simulink model "FOC_BLDC_HIL"  (R2021a)
settings: Solver=FixedStepDiscrete  StartTime=0.0  StopTime=2  RelTol=1e-3  EnableMultiTasking=on
undefined symbols (not defined in the file): DiscIntNeverNeededParam, Init_angle, J, Kawspeed, Ke, Kspeed, Lsx, Lsy, negVid, negVTm, oversampling, p, posVid, posVTm, Psim, Rs, T_load, Ts, ts_FPGA_clk, ts_FPGA_mdl, Ts_svpwm, Tsp, Vdc, Viq, VTm
libraries: simulink x93, hdlsllib x23, slrealtimeloglib x3
(part 3 of 4)

== system FOC_BLDC_HIL/Field Oriented Control ==
  Wm_ref : Inport
  Mech_Speed : Inport  Port=2
  iabc : Inport  Port=3
  Angle estimation : Subsystem
  Clark and Park Transform : Subsystem
  Current Controller : Subsystem
  Rate Transition1 : RateTransition  OutPortSampleTime=Tsp
  Rate Transition7 : RateTransition  OutPortSampleTime=Ts
  SVPWM : Subsystem
  Speed Controller : Subsystem
  "rpm -> rad/s [mech.]" : Gain  Gain=2*pi/60
  Ta,Tb,Tc : Outport
  wires:
  Speed Controller/1(idq_ref) -> Rate Transition7/1
  Wm_ref/1 -> "rpm -> rad/s [mech.]"/1
  Rate Transition1/1 -> Speed Controller/2(Wm)
  iabc/1 -> Clark and Park Transform/2(iabc)
  Mech_Speed/1 -> Angle estimation/1(Mech_Speed), Rate Transition1/1, Current Controller/3(Wm)
  Current Controller/1(vabc*) -> SVPWM/1(vabc*)
  Rate Transition7/1 -> Current Controller/1(Idq_ref)
  Clark and Park Transform/1(idq) -> Current Controller/2(idq)
  "rpm -> rad/s [mech.]"/1 -> Speed Controller/1(Wm_ref)
  SVPWM/1("Ta,Tb,Tc ") -> Ta,Tb,Tc/1
  Angle estimation/1(angle_el) -> Current Controller/4(Angle_el), Clark and Park Transform/1(angle)

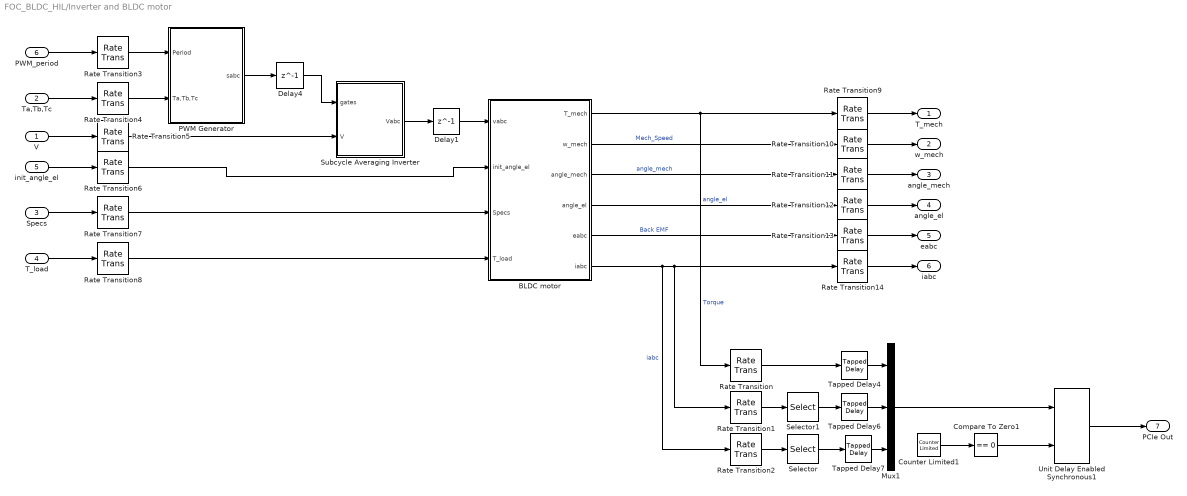
== system FOC_BLDC_HIL/Inverter and BLDC motor ==
  V : Inport
  Ta,Tb,Tc : Inport  Port=2
  Specs : Inport  Port=3
  T_load : Inport  Port=4
  init_angle_el : Inport  Port=5
  PWM_period : Inport  Port=6
  "\tPWM Generator" : Subsystem
  BLDC motor : Subsystem
  Compare To Zero1 : simulink/Logic and Bit Operations/Compare To Zero  relop===  OutDataTypeStr=boolean
  Counter Limited1 : simulink/Sources/Counter Limited  uplimit=49  tsamp=Ts
  Delay1 : Delay  DelayLength=1
  Delay4 : Delay  DelayLength=1
  Mux1 : Mux  Inputs=3
  Rate Transition{,1..2,5..8,10} (8 alike) : RateTransition
  Rate Transition{9,11..14} (5 alike) : RateTransition  OutPortSampleTime=Ts
  Rate Transition3 : RateTransition  OutPortSampleTime=ts_FPGA_clk
  Rate Transition4 : RateTransition  OutPortSampleTime=ts_FPGA_clk
  Selector : Selector  InputPortWidth=3  IndexOptions=Index vector (dialog)  Indices=[2]  OutputSizes=1
  Selector1 : Selector  InputPortWidth=3  IndexOptions=Index vector (dialog)  Indices=[1]  OutputSizes=1
  Subcycle Averaging Inverter : Subsystem
  Tapped Delay4 : simulink/Discrete/Tapped Delay  vinit=0.0  samptime=Ts  NumDelays=50  DelayOrder=Oldest  includeCurrent=off
  Tapped Delay6 : simulink/Discrete/Tapped Delay  vinit=0.0  samptime=Ts  NumDelays=50  DelayOrder=Oldest  includeCurrent=off
  Tapped Delay7 : simulink/Discrete/Tapped Delay  vinit=0.0  samptime=Ts  NumDelays=50  DelayOrder=Oldest  includeCurrent=off
  Unit Delay Enabled Synchronous1 : hdlsllib/Discrete/Unit Delay Enabled Synchronous  InitialCondition=0.0  SampleTime=Ts
      settings: SourceProductName=HDL Coder
  T_mech : Outport
  w_mech : Outport  Port=2
  angle_mech : Outport  Port=3
  angle_el : Outport  Port=4
  eabc : Outport  Port=5
  iabc : Outport  Port=6
  PCIe Out : Outport  Port=7
  wires:
  BLDC motor/3(angle_mech) -> Rate Transition11/1  "angle_mech"
  BLDC motor/5(eabc) -> Rate Transition13/1  "Back EMF"
  Ta,Tb,Tc/1 -> Rate Transition4/1
  PWM_period/1 -> Rate Transition3/1
  "\tPWM Generator"/1("sabc ") -> Delay4/1
  Subcycle Averaging Inverter/1(Vabc) -> Delay1/1
  init_angle_el/1 -> Rate Transition6/1
  Specs/1 -> Rate Transition7/1
  T_load/1 -> Rate Transition8/1
  Delay4/1 -> Subcycle Averaging Inverter/1(gates)
  V/1 -> Rate Transition5/1
  Delay1/1 -> BLDC motor/1(vabc)
  Tapped Delay4/1 -> Mux1/1
  Compare To Zero1/1 -> Unit Delay Enabled Synchronous1/2
  Unit Delay Enabled Synchronous1/1 -> PCIe Out/1
  Mux1/1 -> Unit Delay Enabled Synchronous1/1
  BLDC motor/1(T_mech) -> Rate Transition/1, Rate Transition9/1  "Torque"
  BLDC motor/6(iabc) -> Rate Transition2/1, Rate Transition1/1, Rate Transition14/1  "iabc"
  BLDC motor/4(angle_el) -> Rate Transition12/1  "angle_el"
  BLDC motor/2(w_mech) -> Rate Transition10/1  "Mech_Speed"
  Counter Limited1/1 -> Compare To Zero1/1
  Selector/1 -> Tapped Delay7/1
  Tapped Delay6/1 -> Mux1/2
  Tapped Delay7/1 -> Mux1/3
  Selector1/1 -> Tapped Delay6/1
  Rate Transition2/1 -> Selector/1
  Rate Transition1/1 -> Selector1/1
  Rate Transition/1 -> Tapped Delay4/1
  Rate Transition3/1 -> "\tPWM Generator"/1(Period)
  Rate Transition4/1 -> "\tPWM Generator"/2(Ta,Tb,Tc)
  Rate Transition5/1 -> Subcycle Averaging Inverter/2(V)
  Rate Transition6/1 -> BLDC motor/2(init_angle_el)
  Rate Transition7/1 -> BLDC motor/3(Specs)
  Rate Transition8/1 -> BLDC motor/4(T_load)
  Rate Transition9/1 -> T_mech/1
  Rate Transition10/1 -> w_mech/1
  Rate Transition11/1 -> angle_mech/1
  Rate Transition12/1 -> angle_el/1
  Rate Transition13/1 -> eabc/1
  Rate Transition14/1 -> iabc/1

== system FOC_BLDC_HIL/Motor Specifications ==
  Data Type Conversion11 : DataTypeConversion  OutDataTypeStr=single  RndMeth=Nearest
  Moment of inertia reciprocal : Constant  Value=1/J  SampleTime=-1
  Mux : Mux  Inputs=7
  Number of pole pairs : Constant  Value=p  SampleTime=Ts
  Permanent magnetic flux linkage : Constant  Value=Psim  SampleTime=-1
  Reciprocal : Product  Inputs=/
  Stator Resistance : Constant  Value=Rs  SampleTime=-1
  Stator inductance in d-axis reciprocal : Constant  Value=1/Lsx  SampleTime=-1
  Stator inductance in q-axis reciprocal : Constant  Value=1/Lsy  SampleTime=-1
  Specs : Outport
  wires:
  Stator inductance in q-axis reciprocal/1 -> Mux/7
  Number of pole pairs/1 -> Reciprocal/1, Mux/1
  Stator inductance in d-axis reciprocal/1 -> Mux/6
  Permanent magnetic flux linkage/1 -> Mux/3
  Stator Resistance/1 -> Mux/5
  Mux/1 -> Data Type Conversion11/1
  Data Type Conversion11/1 -> Specs/1
  Moment of inertia reciprocal/1 -> Mux/4
  Reciprocal/1 -> Mux/2

== system FOC_BLDC_HIL/Subsystem1 ==
  Torque : Inport
  Mech_Speed : Inport  Port=2
  angle_mech : Inport  Port=3
  angle_el : Inport  Port=4
  Back EMF : Inport  Port=5
  iabc : Inport  Port=6
  tag scope: Angle_el=global, Angle_m=global, Iabc=global, Speed=global, Torque=global, back_emf=global
  wires:
  Torque/1 -> [Torque]
  Mech_Speed/1 -> [Speed]
  Back EMF/1 -> [back_emf]
  angle_mech/1 -> [Angle_m]
  iabc/1 -> [Iabc]
  angle_el/1 -> [Angle_el]

== system FOC_BLDC_HIL/Field Oriented Control/Angle estimation ==
  Mech_Speed : Inport
  Discrete-Time Integrator1 : DiscreteIntegrator  SampleTime=-1  ICPrevOutput=DiscIntNeverNeededParam  ICPrevScaledInput=DiscIntNeverNeededParam
  Initial motor angle : Constant  Value=Init_angle  OutDataTypeStr=single
  Sum4 : Sum  OutDataTypeStr=single
  Wrapped Discrete Time Integrator : Subsystem
  p/2 : Gain  Gain=p
  angle_el : Outport
  wires:
  p/2/1 -> Wrapped Discrete Time Integrator/1(In1)  "electrical_speed"
  Wrapped Discrete Time Integrator/1(Out1) -> Sum4/1
  Mech_Speed/1 -> p/2/1
  Sum4/1 -> angle_el/1  "Electrical_angle"
  Initial motor angle/1 -> Sum4/2

== system FOC_BLDC_HIL/Field Oriented Control/Clark and Park Transform ==
  angle : Inport
  iabc : Inport  Port=2
  Phase advancement : Subsystem  Commented=on
  Sine_Cosine : Trigonometry  Operator=sincos
  "abc -> d/q" : Subsystem
  idq : Outport  VectorParamsAs1DForOutWhenUnconnected=off
  wires:
  Sine_Cosine/1 -> "abc -> d/q"/2(Sin)
  Sine_Cosine/2 -> "abc -> d/q"/3(Cos)
  iabc/1 -> "abc -> d/q"/1(iabc)
  "abc -> d/q"/1(idq) -> idq/1
  angle/1 -> Sine_Cosine/1

== system FOC_BLDC_HIL/Field Oriented Control/Current Controller ==
  Idq_ref : Inport
  idq : Inport  Port=2
  Wm : Inport  Port=3
  Angle_el : Inport  Port=4
  Phase advancement : Subsystem
  Sine_Cosine : Trigonometry  Operator=sincos
  Trapezoidal emf estimator : Subsystem
  "d/q -> abc" : Subsystem
  d/q controller : Subsystem
  vabc* : Outport  VectorParamsAs1DForOutWhenUnconnected=off
  wires:
  Trapezoidal emf estimator/1(Trapezoidal edq) -> d/q controller/3(edq)
  Idq_ref/1 -> d/q controller/1(Idq_ref)
  idq/1 -> d/q controller/2(idq)
  Angle_el/1 -> Trapezoidal emf estimator/2(Angle_el), Phase advancement/1(angle)
  Wm/1 -> Trapezoidal emf estimator/1(Wm)
  Sine_Cosine/1 -> "d/q -> abc"/2(Sin)
  Sine_Cosine/2 -> "d/q -> abc"/3(Cos)
  Phase advancement/1(ph.adv. angle) -> Sine_Cosine/1
  d/q controller/1(vdq) -> "d/q -> abc"/1(vdq)
  "d/q -> abc"/1(vabc) -> vabc*/1

== system FOC_BLDC_HIL/Field Oriented Control/SVPWM ==
  vabc* : Inport
  Application times : Subsystem
  Magnitude Invariant Clark : Subsystem
  On-state times : Subsystem
  Sector selector : Subsystem
  Ts_svpwm : Constant  Value=Ts_svpwm  OutDataTypeStr=single
  Vdc : Constant  Value=Vdc  OutDataTypeStr=single  SampleTime=-1
  XYZ : Subsystem
  "Ta,Tb,Tc " : Outport  VectorParamsAs1DForOutWhenUnconnected=off
  wires:
  Ts_svpwm/1 -> Application times/3(Ts), On-state times/3(Ts), XYZ/3(Ts)
  Sector selector/1(N) -> On-state times/1(N), Application times/1(N)
  Application times/1(T1,T2) -> On-state times/2("T1,T2 ")
  Magnitude Invariant Clark/1(Valphabeta) -> Sector selector/1(Valphabeta), XYZ/2(vAB)
  vabc*/1 -> Magnitude Invariant Clark/1(vabc)
  XYZ/1(XYZ) -> Application times/2(XYZ)
  Vdc/1 -> XYZ/1(VDC)
  On-state times/1(Ta,Tb,Tc) -> "Ta,Tb,Tc "/1

== system FOC_BLDC_HIL/Field Oriented Control/Speed Controller ==
  Wm_ref : Inport
  Wm : Inport  Port=2
  Speed controller : Subsystem
  idq_ref : Outport  VectorParamsAs1DForOutWhenUnconnected=off
  wires:
  Wm_ref/1 -> Speed controller/1(Wm_ref)
  Wm/1 -> Speed controller/2(Wm)
  Speed controller/1(idq_ref) -> idq_ref/1

== system FOC_BLDC_HIL/Inverter and BLDC motor/	PWM Generator ==
  Period : Inport
  Ta,Tb,Tc : Inport  Port=2
  Demux : Demux  Outputs=3
  Logical Operator : Logic  Operator=NOT  AllPortsSameDT=off  OutDataTypeStr=boolean
  Logical Operator1 : Logic  Operator=NOT  AllPortsSameDT=off  OutDataTypeStr=boolean
  Logical Operator2 : Logic  Operator=NOT  AllPortsSameDT=off  OutDataTypeStr=boolean
  Mux : Mux  Inputs=6
  Relational Operator1 : RelationalOperator  Operator=>  OutDataTypeStr=boolean  RndMeth=Nearest
  Relational Operator2 : RelationalOperator  Operator=>  OutDataTypeStr=boolean  RndMeth=Nearest
  Relational Operator3 : RelationalOperator  Operator=>  OutDataTypeStr=boolean  RndMeth=Nearest
  Unit Delay : UnitDelay  SampleTime=-1  HasFrameUpgradeWarning=on
  carrier_wave1 : Subsystem
  "sabc " : Outport  VectorParamsAs1DForOutWhenUnconnected=off
  wires:
  Unit Delay/1 -> Relational Operator3/1, Relational Operator2/1, Relational Operator1/1  "Counter"
  Relational Operator1/1 -> Logical Operator/1, Mux/1  "A"
  Relational Operator2/1 -> Mux/3, Logical Operator1/1  "B"
  Logical Operator1/1 -> Mux/4  "B_"
  Relational Operator3/1 -> Mux/5, Logical Operator2/1  "C"
  Logical Operator2/1 -> Mux/6  "C_"
  Logical Operator/1 -> Mux/2  "A_"
  Mux/1 -> "sabc "/1  "G"
  Demux/1 -> Relational Operator1/2  "A_comp"
  Demux/2 -> Relational Operator2/2  "B_comp"
  Demux/3 -> Relational Operator3/2  "C_comp"
  Ta,Tb,Tc/1 -> Demux/1
  Period/1 -> carrier_wave1/1(PWM_period)
  carrier_wave1/1(counter) -> Unit Delay/1

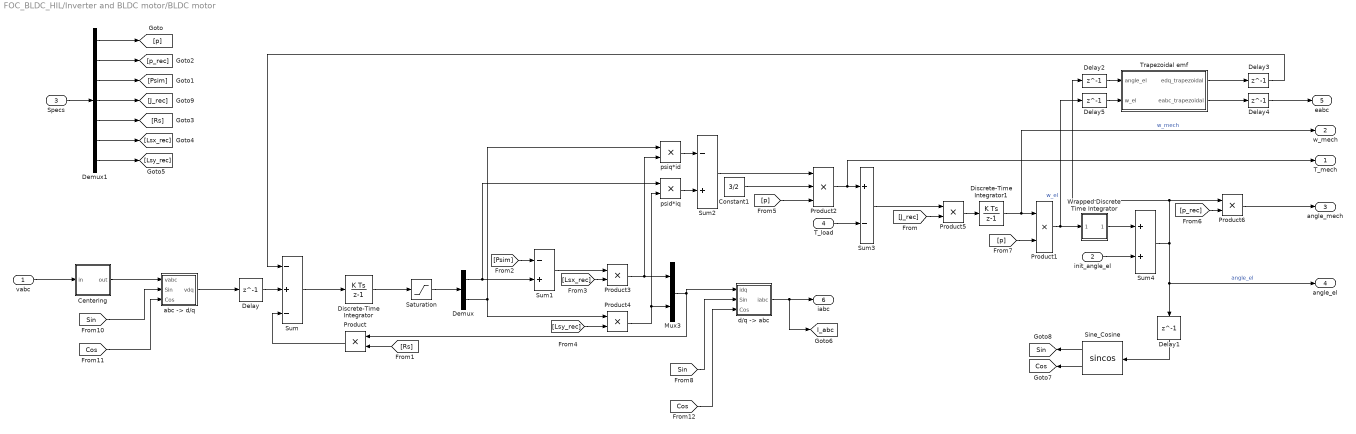
== system FOC_BLDC_HIL/Inverter and BLDC motor/BLDC motor ==
  vabc : Inport
  init_angle_el : Inport  Port=2
  Specs : Inport  Port=3
  T_load : Inport  Port=4
  Centering : Subsystem
  Constant1 : Constant  Value=3/2  OutDataTypeStr=single  SampleTime=-1
  Delay{,1..5} (6 alike) : Delay  DelayLength=1
  Demux : Demux  Outputs=2
  Demux1 : Demux  Outputs=7
  Discrete-Time Integrator : DiscreteIntegrator  InitialCondition=[Psim 0]'  SampleTime=-1  ICPrevOutput=DiscIntNeverNeededParam  ICPrevScaledInput=DiscIntNeverNeededParam
  Discrete-Time Integrator1 : DiscreteIntegrator  SampleTime=-1  ICPrevOutput=DiscIntNeverNeededParam  ICPrevScaledInput=DiscIntNeverNeededParam
  Mux3 : Mux  Inputs=2
  Product{,1,3..6} (6 alike) : Product
  Product2 : Product  Inputs=3
  Saturation : Saturate  UpperLimit=2*[Psim Psim]'  LowerLimit=-2*[Psim Psim]'
  Sine_Cosine : Trigonometry  Operator=sincos
  Sum : Sum  Inputs=-+-
  Sum1 : Sum  Inputs=-+
  Sum2 : Sum  Inputs=-+
  Sum3 : Sum  Inputs=+-
  Sum4 : Sum  OutDataTypeStr=single
  Trapezoidal emf : Subsystem
  Wrapped Discrete Time Integrator : Subsystem
  "abc -> d/q" : Subsystem
  "d/q -> abc" : Subsystem
  psid*iq : Product
  psiq*id : Product
  T_mech : Outport  VectorParamsAs1DForOutWhenUnconnected=off
  w_mech : Outport  Port=2  VectorParamsAs1DForOutWhenUnconnected=off
  angle_mech : Outport  Port=3  VectorParamsAs1DForOutWhenUnconnected=off
  angle_el : Outport  Port=4  VectorParamsAs1DForOutWhenUnconnected=off
  eabc : Outport  Port=5  VectorParamsAs1DForOutWhenUnconnected=off
  iabc : Outport  Port=6  VectorParamsAs1DForOutWhenUnconnected=off
  tag scope: Cos=global, I_abc=global, Sin=global
  wires:
  Product4/1 -> psid*iq/2, Mux3/2
  [Psim] -> Sum1/1
  psiq*id/1 -> Sum2/1
  Product3/1 -> Mux3/1, psiq*id/2
  Mux3/1 -> "d/q -> abc"/1(idq), Product/1
  psid*iq/1 -> Sum2/2
  Sum/1 -> Discrete-Time Integrator/1
  T_load/1 -> Sum3/2
  Demux/1 -> Sum1/2, psid*iq/1
  Sum1/1 -> Product3/1
  Product5/1 -> Discrete-Time Integrator1/1
  Demux/2 -> Product4/1, psiq*id/1
  Discrete-Time Integrator1/1 -> w_mech/1, Product1/1  "w_mech"
  Product2/1 -> T_mech/1, Sum3/1
  Discrete-Time Integrator/1 -> Saturation/1
  Product6/1 -> angle_mech/1
  Saturation/1 -> Demux/1
  Wrapped Discrete Time Integrator/1(Out1) -> Sum4/1
  init_angle_el/1 -> Sum4/2
  Sum4/1 -> Product6/1, Delay2/1, Delay1/1, angle_el/1  "angle_el"
  Product1/1 -> Wrapped Discrete Time Integrator/1(In1), Delay5/1  "w_el"
  Specs/1 -> Demux1/1
  Product/1 -> Sum/3
  [Rs] -> Product/2
  [Lsx_rec] -> Product3/2
  [Lsy_rec] -> Product4/2
  Sum2/1 -> Product2/1
  Constant1/1 -> Product2/2
  [p] -> Product2/3
  Sum3/1 -> Product5/1
  [J_rec] -> Product5/2
  [p] -> Product1/2
  Demux1/1 -> [p]
  Demux1/5 -> [Rs]
  Demux1/6 -> [Lsx_rec]
  Demux1/7 -> [Lsy_rec]
  Demux1/2 -> [p_rec]
  Trapezoidal emf/1(edq_trapezoidal) -> Delay3/1
  Trapezoidal emf/2(eabc_trapezoidal) -> Delay4/1
  Sine_Cosine/2 -> [Cos]
  Sine_Cosine/1 -> [Sin]
  vabc/1 -> Centering/1(in)
  Centering/1(out) -> "abc -> d/q"/1(vabc)
  [Sin] -> "abc -> d/q"/2(Sin)
  [Cos] -> "abc -> d/q"/3(Cos)
  "abc -> d/q"/1(vdq) -> Delay/1
  "d/q -> abc"/1(iabc) -> [I_abc], iabc/1
  [Sin] -> "d/q -> abc"/2(Sin)
  [Cos] -> "d/q -> abc"/3(Cos)
  Delay/1 -> Sum/2
  Delay1/1 -> Sine_Cosine/1
  Delay2/1 -> Trapezoidal emf/1(angle_el)
  Delay3/1 -> Sum/1
  Delay4/1 -> eabc/1
  Delay5/1 -> Trapezoidal emf/2(w_el)
  Demux1/4 -> [J_rec]
  Demux1/3 -> [Psim]
  [p_rec] -> Product6/2

== system FOC_BLDC_HIL/Inverter and BLDC motor/Subcycle Averaging Inverter ==
  gates : Inport
  V : Inport  Port=2
  Constant2 : Constant  Value=0  OutDataTypeStr=uint32  SampleTime=1e-6
  Constant3 : Constant  Value=false  SampleTime=-1
  Gain : Gain  Gain=-1
  Inverter (2-Level HDL w faults) : Subsystem  mask{rSnub=10000, rSwitch=0.001, vfSwitch=0, rDiode=0.001, vfDiode=0.8}
      mask prompts: rSnub "Snubber Resistance (Ohms)"; rSwitch "Switch Resistance (Ohms)"; vfSwitch "Switch Forward Voltage (V)"; rDiode "Diode Resistance (Ohms)"; vfDiode "Diode Forward Voltage (V)"
  Selector : Selector  InputPortWidth=3  IndexOptions=Index vector (dialog)  Indices=[1 2]  OutputSizes=1
  Terminator : Terminator
  Terminator1 : Terminator
  Vabc : Outport
  wires:
  Gain/1 -> Inverter (2-Level HDL w faults)/4(V_minus)
  Constant3/1 -> Inverter (2-Level HDL w faults)/6(ideal_switch_flag)
  V/1 -> Inverter (2-Level HDL w faults)/3(V_plus), Gain/1
  Constant2/1 -> Inverter (2-Level HDL w faults)/5(Fault_Word)
  Inverter (2-Level HDL w faults)/3(IDC) -> Terminator1/1
  [I_abc] -> Inverter (2-Level HDL w faults)/2(Iout)
  gates/1 -> Inverter (2-Level HDL w faults)/1(Gates)
  Inverter (2-Level HDL w faults)/1(Vll) -> Selector/1
  Inverter (2-Level HDL w faults)/2(V) -> Vabc/1
  Selector/1 -> Terminator/1

== system FOC_BLDC_HIL/Field Oriented Control/Angle estimation/Wrapped Discrete Time Integrator ==
  In1 : Inport
  Add1 : Sum  Inputs=+++
  Compare To Constant1 : simulink/Logic and Bit Operations/Compare To Constant  relop=>=  const=2*pi  OutDataTypeStr=boolean
  Compare To Constant2 : simulink/Logic and Bit Operations/Compare To Constant  relop=<  const=0  OutDataTypeStr=boolean
  Constant2 : Constant  Value=-2*pi  OutDataTypeStr=single  SampleTime=-1
  Constant3 : Constant  Value=2*pi  OutDataTypeStr=single  SampleTime=-1
  Constant5 : Constant  Value=0  OutDataTypeStr=single  SampleTime=-1
  Gain : Gain  Gain=Ts
  Switch2 : Switch  Criteria=u2 ~= 0
  Switch3 : Switch  Criteria=u2 ~= 0
  Unit Delay : UnitDelay  SampleTime=-1  HasFrameUpgradeWarning=on
  Out1 : Outport  VectorParamsAs1DForOutWhenUnconnected=off
  wires:
  Add1/1 -> Unit Delay/1
  In1/1 -> Gain/1
  Unit Delay/1 -> Out1/1, Add1/1, Compare To Constant2/1, Compare To Constant1/1
  Compare To Constant1/1 -> Switch3/2
  Compare To Constant2/1 -> Switch2/2
  Constant3/1 -> Switch2/1
  Constant5/1 -> Switch2/3
  Switch2/1 -> Switch3/3
  Constant2/1 -> Switch3/1
  Switch3/1 -> Add1/3
  Gain/1 -> Add1/2

== system FOC_BLDC_HIL/Field Oriented Control/Clark and Park Transform/Phase advancement ==
  angle : Inport
  Discrete Derivative : simulink/Discrete/Discrete Derivative  gainval=1.0  ICPrevScaledInput=0.0  OutMin=[]  OutMax=[]  OutDataType=fixdt(1, 16)  OutScaling=2^-10  DoSatur=off
  Sum2 : Sum
  Ts : Gain  Gain=Ts
  ph.adv. angle : Outport  VectorParamsAs1DForOutWhenUnconnected=off
  wires:
  Sum2/1 -> ph.adv. angle/1
  Ts/1 -> Sum2/1
  angle/1 -> Discrete Derivative/1, Sum2/2
  Discrete Derivative/1 -> Ts/1

== system FOC_BLDC_HIL/Field Oriented Control/Clark and Park Transform/abc -> d//q ==
  iabc : Inport
  Sin : Inport  Port=2
  Cos : Inport  Port=3
  Demux : Demux  Outputs=3
  Gain : Gain  Gain=sqrt(3/2)
  Gain1 : Gain  Gain=sqrt(1/2)
  Gain2 : Gain  Gain=-1  OutDataTypeStr=single
  Mux2 : Mux  Inputs=2
  Product{,1..3} (4 alike) : Product
  Subtract : Sum  Inputs=+-
  Subtract1 : Sum
  Sum : Sum  Inputs=+|-
  idq : Outport  VectorParamsAs1DForOutWhenUnconnected=off
  wires:
  iabc/1 -> Demux/1
  Demux/1 -> Gain/1
  Demux/2 -> Sum/1
  Demux/3 -> Sum/2
  Gain/1 -> Product2/1, Product/1  "Alpha"
  Mux2/1 -> idq/1
  Sum/1 -> Gain1/1
  Cos/1 -> Product3/2, Product/2
  Gain1/1 -> Product3/1, Product1/1  "Beta"
  Sin/1 -> Gain2/1
  Product/1 -> Subtract/1
  Product1/1 -> Subtract/2
  Subtract/1 -> Mux2/1
  Product2/1 -> Subtract1/1
  Product3/1 -> Subtract1/2
  Subtract1/1 -> Mux2/2
  Gain2/1 -> Product1/2, Product2/2

== system FOC_BLDC_HIL/Field Oriented Control/Current Controller/Phase advancement ==
  angle : Inport
  Discrete Derivative : simulink/Discrete/Discrete Derivative  gainval=1.0  ICPrevScaledInput=0.0  OutMin=[]  OutMax=[]  OutDataType=fixdt(1, 16)  OutScaling=2^-10  DoSatur=off
  Sum2 : Sum
  Ts : Gain  Gain=Ts
  ph.adv. angle : Outport  VectorParamsAs1DForOutWhenUnconnected=off
  wires:
  Sum2/1 -> ph.adv. angle/1
  Ts/1 -> Sum2/1
  angle/1 -> Discrete Derivative/1, Sum2/2
  Discrete Derivative/1 -> Ts/1

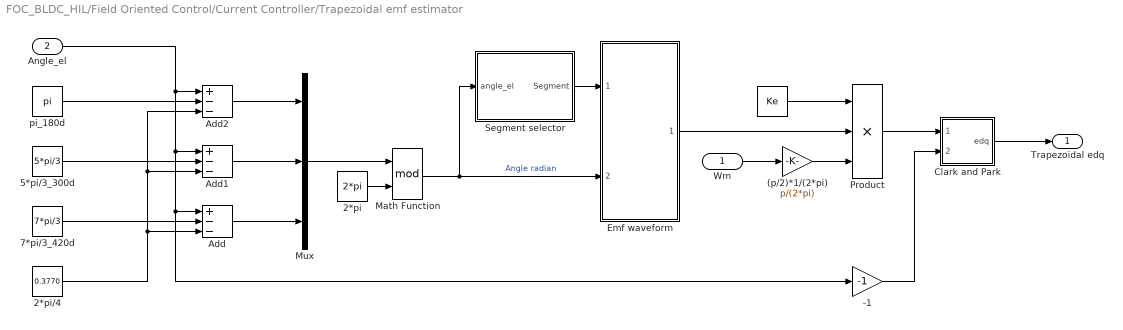
== system FOC_BLDC_HIL/Field Oriented Control/Current Controller/Trapezoidal emf estimator ==
  Wm : Inport
  Angle_el : Inport  Port=2
  "  " : Constant  Value=Ke  OutDataTypeStr=single  SampleTime=-1
  "  Add2" : Sum  Inputs=+--
  " Add1 " : Sum  Inputs=+--
  (p/2)*1/(2*pi) : Gain  Gain=p/(2*pi)
  -1 : Gain  Gain=-1
  2*pi : Constant  Value=2*pi  OutDataTypeStr=single  SampleTime=-1
  2*pi/4 : Constant  Value=0.3770  OutDataTypeStr=single  SampleTime=-1
  5*pi/3_300d : Constant  Value=5*pi/3  OutDataTypeStr=single  SampleTime=-1
  7*pi/3_420d : Constant  Value=7*pi/3  OutDataTypeStr=single  SampleTime=-1
  "Add " : Sum  Inputs=+--
  Clark and Park : Subsystem
  Emf waveform : Subsystem
  Math Function : Math  Operator=mod  SignedPower=on  SaturateOnIntegerOverflow=on
  Mux : Mux  Inputs=3
  Product : Product  Inputs=3
  Segment selector : Subsystem
  pi_180d : Constant  Value=pi  OutDataTypeStr=single  SampleTime=-1
  Trapezoidal edq : Outport  VectorParamsAs1DForOutWhenUnconnected=off
  wires:
  Math Function/1 -> Segment selector/1(angle_el), Emf waveform/2(angle_el)  "Angle radian"
  2*pi/1 -> Math Function/2
  Segment selector/1(Segment) -> Emf waveform/1(Segment)
  " Add1 "/1 -> Mux/2
  5*pi/3_300d/1 -> " Add1 "/2
  "Add "/1 -> Mux/3
  7*pi/3_420d/1 -> "Add "/2
  "  "/1 -> Product/1
  Emf waveform/1(Emf waveform) -> Product/2
  Product/1 -> Clark and Park/1(eabc)
  Wm/1 -> (p/2)*1/(2*pi)/1
  Mux/1 -> Math Function/1
  (p/2)*1/(2*pi)/1 -> Product/3
  -1/1 -> Clark and Park/2(angle)
  Clark and Park/1(edq) -> Trapezoidal edq/1
  "  Add2"/1 -> Mux/1
  pi_180d/1 -> "  Add2"/2
  2*pi/4/1 -> "Add "/3, " Add1 "/3, "  Add2"/3
  Angle_el/1 -> -1/1, "Add "/1, " Add1 "/1, "  Add2"/1

== system FOC_BLDC_HIL/Field Oriented Control/Current Controller/d//q -> abc ==
  vdq : Inport
  Sin : Inport  Port=2
  Cos : Inport  Port=3
  Demux : Demux  Outputs=2
  Gain : Gain  Gain=sqrt(2/3)
  Gain1 : Gain  Gain=-sqrt(1/6)
  Gain2 : Gain  Gain=sqrt(1/2)
  Gain3 : Gain  Gain=sqrt(1/6)
  Gain4 : Gain  Gain=sqrt(1/2)
  Mux2 : Mux  Inputs=3
  Product{,1..3} (4 alike) : Product
  Sum : Sum  Inputs=+|-
  Sum1 : Sum  Inputs=+|+
  Sum2 : Sum  Inputs=+|+
  Sum3 : Sum  Inputs=-|-
  vabc : Outport  VectorParamsAs1DForOutWhenUnconnected=off
  wires:
  vdq/1 -> Demux/1
  Mux2/1 -> vabc/1
  Demux/1 -> Product2/1, Product/1
  Demux/2 -> Product3/1, Product1/1
  Cos/1 -> Product3/2, Product/2
  Sin/1 -> Product2/2, Product1/2
  Product/1 -> Sum/1
  Product1/1 -> Sum/2
  Product3/1 -> Sum1/2
  Product2/1 -> Sum1/1
  Sum/1 -> Gain1/1, Gain3/1, Gain/1  "Alpha"
  Gain/1 -> Mux2/1  "a"
  Gain1/1 -> Sum2/1
  Gain2/1 -> Sum2/2
  Sum1/1 -> Gain4/1, Gain2/1
  Sum2/1 -> Mux2/2  "b"
  Gain3/1 -> Sum3/1
  Gain4/1 -> Sum3/2
  Sum3/1 -> Mux2/3  "c"

== system FOC_BLDC_HIL/Field Oriented Control/Current Controller/d//q controller ==
  Idq_ref : Inport
  idq : Inport  Port=2
  edq : Inport  Port=3
  Demux : Demux  Outputs=2
  Demux1 : Demux  Outputs=2
  Demux2 : Demux  Outputs=2
  Mux1 : Mux  Inputs=2
  Sum1 : Sum  Inputs=+-
  Sum3 : Sum  Inputs=+-
  id controller : Subsystem
  iq controller : Subsystem
  vdq : Outport  VectorParamsAs1DForOutWhenUnconnected=off
  wires:
  Demux/1 -> id controller/2(ed)
  id controller/1(vd) -> Mux1/1
  Demux2/2 -> Sum3/2
  Demux1/2 -> Sum3/1
  Demux/2 -> iq controller/2(eq)
  Sum3/1 -> iq controller/1(iq_error)
  iq controller/1(vq) -> Mux1/2
  Mux1/1 -> vdq/1
  Demux2/1 -> Sum1/2
  Demux1/1 -> Sum1/1
  Sum1/1 -> id controller/1(id_error)
  edq/1 -> Demux/1
  idq/1 -> Demux2/1
  Idq_ref/1 -> Demux1/1

== system FOC_BLDC_HIL/Field Oriented Control/SVPWM/Application times ==
  N : Inport
  XYZ : Inport  Port=2
  Ts : Inport  Port=3
  " " : Gain  Gain=-1
  "  " : Gain  Gain=-1
  "    " : Gain  Gain=-1
  Add : Sum
  Add1 : Sum  Inputs=+--
  Demux : Demux  Outputs=3
  Divide : Product  Inputs=**/
  Divide1 : Product  Inputs=**/
  Multiport Switch : MultiPortSwitch  Inputs=6  DiagnosticForDefault=None
  Multiport Switch1 : MultiPortSwitch  Inputs=6  DiagnosticForDefault=None
  Mux : Mux  Inputs=2
  Switch : Switch
  Switch1 : Switch  Criteria=u2 > Threshold
  T1,T2 : Outport  VectorParamsAs1DForOutWhenUnconnected=off
  wires:
  Demux/2 -> Multiport Switch/3, Multiport Switch1/2, "  "/1
  Demux/3 -> Multiport Switch/2, Multiport Switch1/5, "    "/1
  "    "/1 -> Multiport Switch/4, Multiport Switch1/7
  "  "/1 -> Multiport Switch/7, Multiport Switch1/6
  " "/1 -> Multiport Switch/5, Multiport Switch1/3
  Multiport Switch1/1 -> Switch1/1, Divide1/1, Add/2, Add1/3
  Mux/1 -> T1,T2/1
  Switch/1 -> Mux/1
  Switch1/1 -> Mux/2
  Add/1 -> Divide/3, Divide1/3
  Ts/1 -> Divide1/2, Add1/1, Divide/2
  Multiport Switch/1 -> Add1/2, Add/1, Divide/1, Switch/1
  Divide/1 -> Switch/3
  Add1/1 -> Switch1/2, Switch/2
  Divide1/1 -> Switch1/3
  Demux/1 -> Multiport Switch/6, Multiport Switch1/4, " "/1
  XYZ/1 -> Demux/1
  N/1 -> Multiport Switch1/1, Multiport Switch/1

== system FOC_BLDC_HIL/Field Oriented Control/SVPWM/Magnitude Invariant Clark ==
  vabc : Inport
  "    " : Gain  Gain=sqrt(3)/2
  "     " : Gain  Gain=sqrt(3)/2
  2/3 : Gain  Gain=2/3
  Add1 : Sum  Inputs=+-
  Demux1 : Demux  Outputs=3
  Gain : Gain  Gain=1/2
  Gain1 : Gain  Gain=1/2
  Mux2 : Mux  Inputs=2
  Sum : Sum  Inputs=+--
  Valphabeta : Outport  VectorParamsAs1DForOutWhenUnconnected=off
  wires:
  Demux1/2 -> Gain/1, "     "/1
  Demux1/3 -> Gain1/1, "    "/1
  vabc/1 -> Demux1/1
  "    "/1 -> Add1/2
  "     "/1 -> Add1/1
  Mux2/1 -> 2/3/1
  Add1/1 -> Mux2/2  "Vbeta"
  2/3/1 -> Valphabeta/1
  Gain1/1 -> Sum/3
  Gain/1 -> Sum/2
  Demux1/1 -> Sum/1
  Sum/1 -> Mux2/1  "Valpha"

== system FOC_BLDC_HIL/Field Oriented Control/SVPWM/On-state times ==
  N : Inport
  "T1,T2 " : Inport  Port=2
  Ts : Inport  Port=3
  1/2 : Gain  Gain=1/2
  1/2 also : Gain  Gain=1/2
  1/4 : Gain  Gain=1/4
  Add : Sum  Inputs=+--
  Add1 : Sum
  Add2 : Sum
  Demux2 : Demux  Outputs=2
  Multiport Switch : MultiPortSwitch  Inputs=6  DiagnosticForDefault=None
  Multiport Switch1 : MultiPortSwitch  Inputs=6  DiagnosticForDefault=None
  Multiport Switch2 : MultiPortSwitch  Inputs=6  DiagnosticForDefault=None
  Mux : Mux  Inputs=3
  Ta,Tb,Tc : Outport  VectorParamsAs1DForOutWhenUnconnected=off
  wires:
  "T1,T2 "/1 -> Demux2/1
  Ts/1 -> Add/1
  Demux2/1 -> Add/2, 1/2/1
  Demux2/2 -> Add/3, 1/2 also/1
  Add/1 -> 1/4/1
  1/2/1 -> Add1/2
  1/4/1 -> Add1/1, Multiport Switch2/7, Multiport Switch2/5, Multiport Switch1/6, Multiport Switch1/2, Multiport Switch/4, Multiport Switch/3
  Add1/1 -> Add2/1, Multiport Switch/7, Multiport Switch/2, Multiport Switch2/6, Multiport Switch2/3, Multiport Switch1/5, Multiport Switch1/4
  1/2 also/1 -> Add2/2
  Add2/1 -> Multiport Switch1/3, Multiport Switch/6, Multiport Switch/5, Multiport Switch1/7, Multiport Switch2/2, Multiport Switch2/4
  Multiport Switch1/1 -> Mux/2
  Multiport Switch2/1 -> Mux/3
  Multiport Switch/1 -> Mux/1
  Mux/1 -> Ta,Tb,Tc/1
  N/1 -> Multiport Switch2/1, Multiport Switch1/1, Multiport Switch/1

== system FOC_BLDC_HIL/Field Oriented Control/SVPWM/Sector selector ==
  Valphabeta : Inport
  1/2 : Gain  Gain=1/2
  2 : Gain  Gain=2
  4 : Gain  Gain=4
  Add : Sum  Inputs=+++
  Add1 : Sum  Inputs=+-
  Add2 : Sum  Inputs=--
  Compare To Constant : simulink/Logic and Bit Operations/Compare To Constant  relop=>=  const=0  OutDataTypeStr=boolean
  Compare To Constant1 : simulink/Logic and Bit Operations/Compare To Constant  relop=>  const=0  OutDataTypeStr=boolean  ZeroCross=off
  Compare To Constant2 : simulink/Logic and Bit Operations/Compare To Constant  relop=>  const=0  OutDataTypeStr=boolean  ZeroCross=off
  Demux : Demux  Outputs=2
  Saturation : Saturate  UpperLimit=6  LowerLimit=1  RndMeth=Ceiling
  sqrt(3)/2 : Gain  Gain=sqrt(3)/2
  N : Outport  VectorParamsAs1DForOutWhenUnconnected=off
  wires:
  Add1/1 -> Compare To Constant1/1
  Compare To Constant2/1 -> 4/1
  Add/1 -> Saturation/1
  Add2/1 -> Compare To Constant2/1
  Compare To Constant1/1 -> 2/1
  Demux/1 -> sqrt(3)/2/1
  Valphabeta/1 -> Demux/1
  2/1 -> Add/1
  4/1 -> Add/2
  Compare To Constant/1 -> Add/3
  sqrt(3)/2/1 -> Add2/1, Add1/1
  Demux/2 -> Compare To Constant/1, 1/2/1
  1/2/1 -> Add1/2, Add2/2
  Saturation/1 -> N/1

== system FOC_BLDC_HIL/Field Oriented Control/SVPWM/XYZ ==
  VDC : Inport
  vAB : Inport  Port=2
  Ts : Inport  Port=3
  3/2 : Gain  Gain=3/2
  Add : Sum
  Add1 : Sum  Inputs=+-
  Demux1 : Demux  Outputs=2
  Mux : Mux  Inputs=3
  X : Product  Inputs=**/
  Y : Product  Inputs=**/
  Z : Product  Inputs=**/
  sqrt(3) : Gain  Gain=sqrt(3)
  sqrt(3)/2 : Gain  Gain=sqrt(3)/2
  XYZ : Outport  VectorParamsAs1DForOutWhenUnconnected=off
  wires:
  Z/1 -> Mux/3
  X/1 -> Mux/1
  vAB/1 -> Demux1/1
  VDC/1 -> X/3, Y/3, Z/3
  Ts/1 -> X/2, Y/2, Z/2
  Demux1/2 -> sqrt(3)/1, sqrt(3)/2/1
  sqrt(3)/2/1 -> Add/1, Add1/1
  3/2/1 -> Add1/2, Add/2
  Demux1/1 -> 3/2/1
  Add/1 -> Y/1
  Add1/1 -> Z/1
  Y/1 -> Mux/2
  sqrt(3)/1 -> X/1
  Mux/1 -> XYZ/1

== system FOC_BLDC_HIL/Field Oriented Control/Speed Controller/Speed controller ==
  Wm_ref : Inport
  Wm : Inport  Port=2
  Current reference generator : Subsystem
  Discrete-Time Integrator : DiscreteIntegrator  SampleTime=Tsp  ICPrevOutput=DiscIntNeverNeededParam  ICPrevScaledInput=DiscIntNeverNeededParam
  Kawspeed : Gain  Gain=Kawspeed
  Kspeed : Gain  Gain=Kspeed
  Kspeed/Tauspeed : Gain  Gain=Kspeed/Tauspeed
  Subtract : Sum  Inputs=+-
  Subtract1 : Sum  Inputs=+-
  Sum1 : Sum  Inputs=+-
  T* : Sum
  Torque calculation : Subsystem
  idq_ref : Outport  VectorParamsAs1DForOutWhenUnconnected=off
  wires:
  Wm_ref/1 -> Sum1/1
  Current reference generator/1(idq_ref) -> idq_ref/1, Torque calculation/1(idq_ref)
  Subtract1/1 -> Kawspeed/1
  Kawspeed/1 -> Subtract/2
  Sum1/1 -> Kspeed/1, Subtract/1
  Kspeed/Tauspeed/1 -> Discrete-Time Integrator/1
  Discrete-Time Integrator/1 -> T*/2
  Kspeed/1 -> T*/1
  Torque calculation/1(Tmax) -> Subtract1/2
  Subtract/1 -> Kspeed/Tauspeed/1
  T*/1 -> Current reference generator/1(T*), Subtract1/1
  Wm/1 -> Sum1/2

== system FOC_BLDC_HIL/Inverter and BLDC motor/	PWM Generator/carrier_wave1 ==
  PWM_period : Inport
  Abs1 : Abs
  Bitwise Operator1 : simulink/Logic and Bit Operations/Bitwise Operator  logicop=OR  UseBitMask=off  NumInputPorts=2  BitMask=bin2dec('11011001')  BitMaskRealWorld=Stored Integer
  Constant : Constant  OutDataTypeStr=boolean  SampleTime=-1
  HDL Counter : hdlsllib/Sources/HDL Counter  CountType=Free running  CountInit=0  CountStep=1  CountMax=25  CountFromType=Initial value  CountFrom=0  CountResetPort=on  CountLoadPort=off  CountEnbPort=on  CountDirPort=off  CountHitOutputPort=off  CountDataType=Unsigned  CountWordLen=32  CountFracLen=0  CountSampTime=1
  Multiply : Gain  Gain=2
  NOT : Logic  Operator=NOT  AllPortsSameDT=off  OutDataTypeStr=boolean
  Relational Operator : RelationalOperator  OutDataTypeStr=boolean  RndMeth=Simplest
  Sum : Sum  Inputs=+-  OutDataTypeStr=int32
  counter : Outport
  wires:
  PWM_period/1 -> Sum/2, Multiply/1
  Relational Operator/1 -> Bitwise Operator1/1
  NOT/1 -> Bitwise Operator1/2
  Sum/1 -> Abs1/1
  HDL Counter/1 -> Sum/1, Relational Operator/1
  Multiply/1 -> Relational Operator/2
  Bitwise Operator1/1 -> HDL Counter/1
  Abs1/1 -> counter/1
  Constant/1 -> NOT/1, HDL Counter/2

== system FOC_BLDC_HIL/Inverter and BLDC motor/BLDC motor/Centering ==
  in : Inport
  1/3 : Gain  Gain=1/3
  Demux1 : Demux  Outputs=3
  Mux2 : Mux  Inputs=3
  Sum : Sum  Inputs=+-
  Sum1 : Sum  Inputs=+-
  Sum2 : Sum  Inputs=+++
  Sum3 : Sum  Inputs=+-
  out : Outport  VectorParamsAs1DForOutWhenUnconnected=off
  wires:
  in/1 -> Demux1/1
  Demux1/1 -> Sum/1, Sum2/1
  Demux1/2 -> Sum2/2, Sum1/1
  Demux1/3 -> Sum2/3, Sum3/1
  Sum2/1 -> 1/3/1
  1/3/1 -> Sum3/2, Sum1/2, Sum/2
  Sum1/1 -> Mux2/2
  Sum/1 -> Mux2/1
  Sum3/1 -> Mux2/3
  Mux2/1 -> out/1

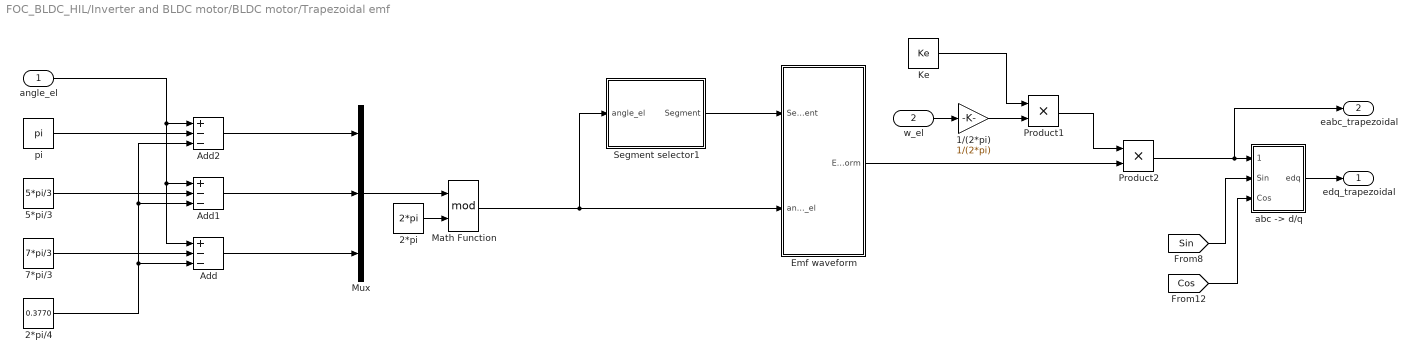
== system FOC_BLDC_HIL/Inverter and BLDC motor/BLDC motor/Trapezoidal emf ==
  angle_el : Inport
  w_el : Inport  Port=2
  "  Add2" : Sum  Inputs=+--  OutDataTypeStr=single
  " Add1 " : Sum  Inputs=+--  OutDataTypeStr=single
  1/(2*pi) : Gain  Gain=1/(2*pi)  OutDataTypeStr=single
  2*pi : Constant  Value=2*pi  OutDataTypeStr=single  SampleTime=-1
  2*pi/4 : Constant  Value=0.3770  OutDataTypeStr=single  SampleTime=-1
  5*pi/3 : Constant  Value=5*pi/3  OutDataTypeStr=single  SampleTime=-1
  7*pi/3 : Constant  Value=7*pi/3  OutDataTypeStr=single  SampleTime=-1
  "Add " : Sum  Inputs=+--  OutDataTypeStr=single
  Emf waveform : Subsystem
  Ke : Constant  Value=Ke  OutDataTypeStr=single  SampleTime=-1
  Math Function : Math  Operator=mod  SignedPower=on  SaturateOnIntegerOverflow=on
  Mux : Mux  Inputs=3
  Product1 : Product
  Product2 : Product
  Segment selector1 : Subsystem
  "abc -> d/q" : Subsystem
  pi : Constant  Value=pi  OutDataTypeStr=single  SampleTime=-1
  edq_trapezoidal : Outport  VectorParamsAs1DForOutWhenUnconnected=off
  eabc_trapezoidal : Outport  Port=2  VectorParamsAs1DForOutWhenUnconnected=off
  wires:
  2*pi/1 -> Math Function/2
  5*pi/3/1 -> " Add1 "/2
  7*pi/3/1 -> "Add "/2
  Ke/1 -> Product1/1
  Emf waveform/1(Emf waveform) -> Product2/2
  w_el/1 -> 1/(2*pi)/1
  Mux/1 -> Math Function/1
  1/(2*pi)/1 -> Product1/2
  angle_el/1 -> "Add "/1, " Add1 "/1, "  Add2"/1
  pi/1 -> "  Add2"/2
  2*pi/4/1 -> "Add "/3, " Add1 "/3, "  Add2"/3
  Math Function/1 -> Segment selector1/1(angle_el), Emf waveform/2(angle_el)
  Product2/1 -> "abc -> d/q"/1(eabc), eabc_trapezoidal/1
  "  Add2"/1 -> Mux/1
  " Add1 "/1 -> Mux/2
  "Add "/1 -> Mux/3
  Segment selector1/1(Segment) -> Emf waveform/1(Segment)
  "abc -> d/q"/1(edq) -> edq_trapezoidal/1
  [Sin] -> "abc -> d/q"/2(Sin)
  [Cos] -> "abc -> d/q"/3(Cos)
  Product1/1 -> Product2/1

== system FOC_BLDC_HIL/Inverter and BLDC motor/BLDC motor/Wrapped Discrete Time Integrator ==
  In1 : Inport
  Add1 : Sum  Inputs=+++
  Compare To Constant1 : simulink/Logic and Bit Operations/Compare To Constant  relop=>=  const=2*pi  OutDataTypeStr=boolean
  Compare To Constant2 : simulink/Logic and Bit Operations/Compare To Constant  relop=<  const=0  OutDataTypeStr=boolean
  Constant2 : Constant  Value=-2*pi  OutDataTypeStr=single  SampleTime=-1
  Constant3 : Constant  Value=2*pi  OutDataTypeStr=single  SampleTime=-1
  Constant5 : Constant  Value=0  OutDataTypeStr=single  SampleTime=-1
  Gain : Gain  Gain=ts_FPGA_mdl
  Switch2 : Switch  Criteria=u2 ~= 0
  Switch3 : Switch  Criteria=u2 ~= 0
  Unit Delay : UnitDelay  SampleTime=-1  HasFrameUpgradeWarning=on
  Out1 : Outport  VectorParamsAs1DForOutWhenUnconnected=off
  wires:
  Add1/1 -> Unit Delay/1
  In1/1 -> Gain/1
  Unit Delay/1 -> Out1/1, Add1/1, Compare To Constant2/1, Compare To Constant1/1
  Compare To Constant1/1 -> Switch3/2
  Compare To Constant2/1 -> Switch2/2
  Constant3/1 -> Switch2/1
  Constant5/1 -> Switch2/3
  Switch2/1 -> Switch3/3
  Constant2/1 -> Switch3/1
  Switch3/1 -> Add1/3
  Gain/1 -> Add1/2

== system FOC_BLDC_HIL/Inverter and BLDC motor/BLDC motor/abc -> d//q ==
  vabc : Inport
  Sin : Inport  Port=2
  Cos : Inport  Port=3
  Demux : Demux  Outputs=3
  Gain : Gain  Gain=sqrt(3/2)
  Gain1 : Gain  Gain=sqrt(1/2)
  Gain2 : Gain  Gain=-1  OutDataTypeStr=single
  Mux2 : Mux  Inputs=2
  Product{,1..3} (4 alike) : Product
  Subtract : Sum  Inputs=+-
  Subtract1 : Sum
  Sum : Sum  Inputs=+|-
  vdq : Outport  VectorParamsAs1DForOutWhenUnconnected=off
  wires:
  vabc/1 -> Demux/1
  Demux/1 -> Gain/1
  Demux/2 -> Sum/1
  Demux/3 -> Sum/2
  Gain/1 -> Product2/1, Product/1  "Alpha"
  Mux2/1 -> vdq/1
  Sum/1 -> Gain1/1
  Cos/1 -> Product3/2, Product/2
  Gain1/1 -> Product3/1, Product1/1  "Beta"
  Sin/1 -> Gain2/1
  Product/1 -> Subtract/1
  Product1/1 -> Subtract/2
  Subtract/1 -> Mux2/1
  Product2/1 -> Subtract1/1
  Product3/1 -> Subtract1/2
  Subtract1/1 -> Mux2/2
  Gain2/1 -> Product1/2, Product2/2

== system FOC_BLDC_HIL/Inverter and BLDC motor/BLDC motor/d//q -> abc ==
  idq : Inport
  Sin : Inport  Port=2
  Cos : Inport  Port=3
  Demux : Demux  Outputs=2
  Gain : Gain  Gain=sqrt(2/3)
  Gain1 : Gain  Gain=-sqrt(1/6)
  Gain2 : Gain  Gain=sqrt(1/2)
  Gain3 : Gain  Gain=sqrt(1/6)
  Gain4 : Gain  Gain=sqrt(1/2)
  Mux2 : Mux  Inputs=3
  Product{,1..3} (4 alike) : Product
  Sum : Sum  Inputs=+|-
  Sum1 : Sum  Inputs=+|+
  Sum2 : Sum  Inputs=+|+
  Sum3 : Sum  Inputs=-|-
  iabc : Outport  VectorParamsAs1DForOutWhenUnconnected=off
  wires:
  idq/1 -> Demux/1
  Mux2/1 -> iabc/1
  Demux/1 -> Product2/1, Product/1
  Demux/2 -> Product3/1, Product1/1
  Cos/1 -> Product3/2, Product/2
  Sin/1 -> Product2/2, Product1/2
  Product/1 -> Sum/1
  Product1/1 -> Sum/2
  Product3/1 -> Sum1/2
  Product2/1 -> Sum1/1
  Sum/1 -> Gain1/1, Gain3/1, Gain/1  "Alpha"
  Gain/1 -> Mux2/1  "a"
  Gain1/1 -> Sum2/1
  Gain2/1 -> Sum2/2
  Sum1/1 -> Gain4/1, Gain2/1
  Sum2/1 -> Mux2/2  "b"
  Gain3/1 -> Sum3/1
  Gain4/1 -> Sum3/2
  Sum3/1 -> Mux2/3  "c"

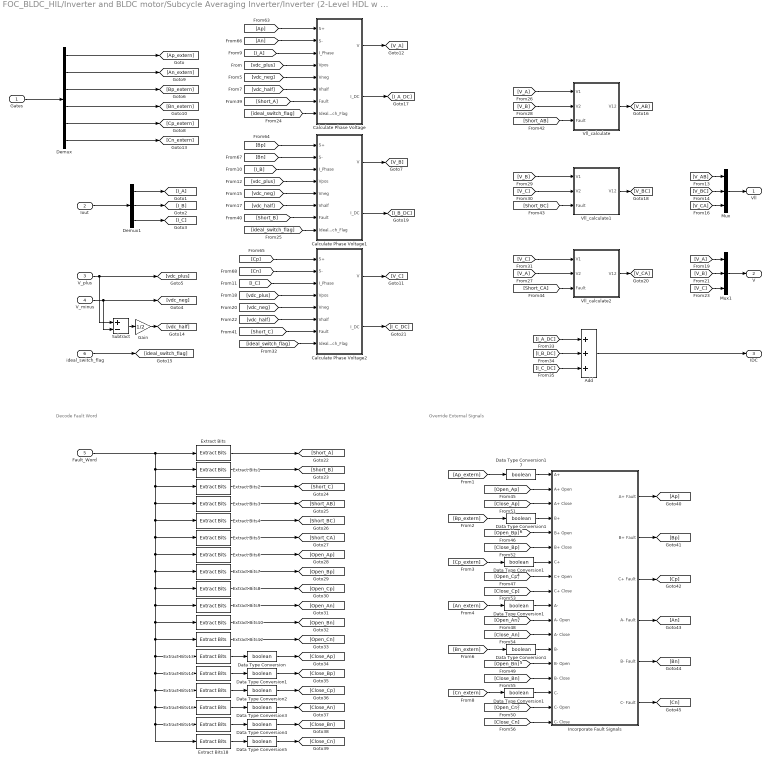
== system FOC_BLDC_HIL/Inverter and BLDC motor/Subcycle Averaging Inverter/Inverter (2-Level HDL w faults) ==
  note: Override External Signals
  note: Decode Fault Word
  Gates : Inport
  Iout : Inport  Port=2
  V_plus : Inport  Port=3
  V_minus : Inport  Port=4
  Fault_Word : Inport  Port=5
  ideal_switch_flag : Inport  Port=6
  Add : Sum  Inputs=+++
  Calculate Phase Voltage : Subsystem
  Calculate Phase Voltage1 : Subsystem
  Calculate Phase Voltage2 : Subsystem
  Data Type Conversion{,1..5,12..17} (12 alike) : DataTypeConversion  OutDataTypeStr=boolean
  Demux : Demux  Outputs=6
  Demux1 : Demux  Outputs=3
  Extract Bits : simulink/Logic and Bit Operations/Extract Bits  bitsToExtract=Range of bits  numBits=8  bitIdxRange=[0]  outScalingMode=Treat bit field as an integer
  Extract Bits1 : simulink/Logic and Bit Operations/Extract Bits  bitsToExtract=Range of bits  numBits=8  bitIdxRange=1  outScalingMode=Treat bit field as an integer
  Extract Bits10 : simulink/Logic and Bit Operations/Extract Bits  bitsToExtract=Range of bits  numBits=8  bitIdxRange=10  outScalingMode=Treat bit field as an integer
  Extract Bits12 : simulink/Logic and Bit Operations/Extract Bits  bitsToExtract=Range of bits  numBits=8  bitIdxRange=11  outScalingMode=Treat bit field as an integer
  Extract Bits13 : simulink/Logic and Bit Operations/Extract Bits  bitsToExtract=Range of bits  numBits=8  bitIdxRange=12  outScalingMode=Treat bit field as an integer
  Extract Bits14 : simulink/Logic and Bit Operations/Extract Bits  bitsToExtract=Range of bits  numBits=8  bitIdxRange=13  outScalingMode=Treat bit field as an integer
  Extract Bits15 : simulink/Logic and Bit Operations/Extract Bits  bitsToExtract=Range of bits  numBits=8  bitIdxRange=14  outScalingMode=Treat bit field as an integer
  Extract Bits16 : simulink/Logic and Bit Operations/Extract Bits  bitsToExtract=Range of bits  numBits=8  bitIdxRange=15  outScalingMode=Treat bit field as an integer
  Extract Bits17 : simulink/Logic and Bit Operations/Extract Bits  bitsToExtract=Range of bits  numBits=8  bitIdxRange=16  outScalingMode=Treat bit field as an integer
  Extract Bits18 : simulink/Logic and Bit Operations/Extract Bits  bitsToExtract=Range of bits  numBits=8  bitIdxRange=17  outScalingMode=Treat bit field as an integer
  Extract Bits2 : simulink/Logic and Bit Operations/Extract Bits  bitsToExtract=Range of bits  numBits=8  bitIdxRange=2  outScalingMode=Treat bit field as an integer
  Extract Bits3 : simulink/Logic and Bit Operations/Extract Bits  bitsToExtract=Range of bits  numBits=8  bitIdxRange=3  outScalingMode=Treat bit field as an integer
  Extract Bits4 : simulink/Logic and Bit Operations/Extract Bits  bitsToExtract=Range of bits  numBits=8  bitIdxRange=4  outScalingMode=Treat bit field as an integer
  Extract Bits5 : simulink/Logic and Bit Operations/Extract Bits  bitsToExtract=Range of bits  numBits=8  bitIdxRange=5  outScalingMode=Treat bit field as an integer
  Extract Bits6 : simulink/Logic and Bit Operations/Extract Bits  bitsToExtract=Range of bits  numBits=8  bitIdxRange=6  outScalingMode=Treat bit field as an integer
  Extract Bits7 : simulink/Logic and Bit Operations/Extract Bits  bitsToExtract=Range of bits  numBits=8  bitIdxRange=7  outScalingMode=Treat bit field as an integer
  Extract Bits8 : simulink/Logic and Bit Operations/Extract Bits  bitsToExtract=Range of bits  numBits=8  bitIdxRange=8  outScalingMode=Treat bit field as an integer
  Extract Bits9 : simulink/Logic and Bit Operations/Extract Bits  bitsToExtract=Range of bits  numBits=8  bitIdxRange=9  outScalingMode=Treat bit field as an integer
  Gain : Gain  Gain=1/2
  Incorporate Fault Signals : Subsystem
  Mux : Mux  Inputs=3
  Mux1 : Mux  Inputs=3
  Subtract : Sum  Inputs=+-
  Vll_calculate : Subsystem
  Vll_calculate1 : Subsystem
  Vll_calculate2 : Subsystem
  Vll : Outport  OutDataTypeStr=single  VectorParamsAs1DForOutWhenUnconnected=off
  V : Outport  Port=2  OutDataTypeStr=single  VectorParamsAs1DForOutWhenUnconnected=off
  IDC : Outport  Port=3  OutDataTypeStr=single  VectorParamsAs1DForOutWhenUnconnected=off
  wires:
  Gates/1 -> Demux/1
  Calculate Phase Voltage/1(V) -> [V_A]
  [V_B] -> Vll_calculate/2(V2)
  [V_A] -> Vll_calculate/1(V1)
  Vll_calculate/1(V12) -> [V_AB]
  Vll_calculate2/1(V12) -> [V_CA]
  Vll_calculate1/1(V12) -> [V_BC]
  Extract Bits9/1 -> [Open_An]
  Extract Bits12/1 -> [Open_Cn]
  [Ap_extern] -> Data Type Conversion17/1
  Incorporate Fault Signals/6(C- Fault) -> [Cn]
  [Open_Cn] -> Incorporate Fault Signals/17(C- Open)
  Incorporate Fault Signals/2(B+ Fault) -> [Bp]
  [Cn_extern] -> Data Type Conversion12/1
  [Close_Bn] -> Incorporate Fault Signals/15(B- Close)
  Incorporate Fault Signals/5(B- Fault) -> [Bn]
  Extract Bits7/1 -> [Open_Bp]
  [Bp_extern] -> Data Type Conversion16/1
  [Close_Cn] -> Incorporate Fault Signals/18(C- Close)
  [Close_Bp] -> Incorporate Fault Signals/6(B+ Close)
  [Open_Bp] -> Incorporate Fault Signals/5(B+ Open)
  [Bn_extern] -> Data Type Conversion15/1
  [Close_An] -> Incorporate Fault Signals/12(A- Close)
  [An_extern] -> Data Type Conversion13/1
  Fault_Word/1 -> Extract Bits/1, Extract Bits1/1, Extract Bits2/1, Extract Bits3/1, Extract Bits4/1, Extract Bits5/1, Extract Bits6/1, Extract Bits7/1, Extract Bits8/1, Extract Bits9/1, Extract Bits10/1, Extract Bits12/1, Extract Bits13/1, Extract Bits14/1, Extract Bits15/1, Extract Bits16/1, Extract Bits18/1, Extract Bits17/1
  Extract Bits6/1 -> [Open_Ap]
  [Open_Ap] -> Incorporate Fault Signals/2(A+ Open)
  Extract Bits8/1 -> [Open_Cp]
  Extract Bits17/1 -> Data Type Conversion4/1
  [Cp_extern] -> Data Type Conversion14/1
  Extract Bits5/1 -> [Short_CA]
  Extract Bits14/1 -> Data Type Conversion1/1
  Extract Bits1/1 -> [Short_B]
  Extract Bits13/1 -> Data Type Conversion/1
  Extract Bits10/1 -> [Open_Bn]
  Incorporate Fault Signals/4(A- Fault) -> [An]
  [Close_Ap] -> Incorporate Fault Signals/3(A+ Close)
  [Open_Cp] -> Incorporate Fault Signals/8(C+ Open)
  Incorporate Fault Signals/1(A+ Fault) -> [Ap]
  Extract Bits4/1 -> [Short_BC]
  Extract Bits18/1 -> Data Type Conversion5/1
  Extract Bits3/1 -> [Short_AB]
  [Open_Bn] -> Incorporate Fault Signals/14(B- Open)
  Extract Bits2/1 -> [Short_C]
  [Open_An] -> Incorporate Fault Signals/11(A- Open)
  Extract Bits15/1 -> Data Type Conversion2/1
  Extract Bits/1 -> [Short_A]
  Incorporate Fault Signals/3(C+ Fault) -> [Cp]
  [Close_Cp] -> Incorporate Fault Signals/9(C+ Close)
  Extract Bits16/1 -> Data Type Conversion3/1
  Iout/1 -> Demux1/1
  Demux1/1 -> [I_A]
  Demux1/2 -> [I_B]
  Demux1/3 -> [I_C]
  [Ap] -> Calculate Phase Voltage/1(S+)
  [I_A] -> Calculate Phase Voltage/3(I_Phase)
  [An] -> Calculate Phase Voltage/2(S-)
  [vdc_plus] -> Calculate Phase Voltage/4(Vpos)
  [vdc_neg] -> Calculate Phase Voltage/5(Vneg)
  [vdc_half] -> Calculate Phase Voltage/6(Vhalf)
  [Short_A] -> Calculate Phase Voltage/7(Fault)
  [Bp] -> Calculate Phase Voltage1/1(S+)
  [Bn] -> Calculate Phase Voltage1/2(S-)
  [I_B] -> Calculate Phase Voltage1/3(I_Phase)
  [vdc_plus] -> Calculate Phase Voltage1/4(Vpos)
  [vdc_neg] -> Calculate Phase Voltage1/5(Vneg)
  [vdc_half] -> Calculate Phase Voltage1/6(Vhalf)
  [Short_B] -> Calculate Phase Voltage1/7(Fault)
  [I_C] -> Calculate Phase Voltage2/3(I_Phase)
  [Cp] -> Calculate Phase Voltage2/1(S+)
  [Cn] -> Calculate Phase Voltage2/2(S-)
  [vdc_plus] -> Calculate Phase Voltage2/4(Vpos)
  [vdc_neg] -> Calculate Phase Voltage2/5(Vneg)
  [Short_C] -> Calculate Phase Voltage2/7(Fault)
  [vdc_half] -> Calculate Phase Voltage2/6(Vhalf)
  Calculate Phase Voltage1/1(V) -> [V_B]
  Calculate Phase Voltage2/1(V) -> [V_C]
  [V_C] -> Vll_calculate2/1(V1)
  [V_A] -> Vll_calculate2/2(V2)
  [V_B] -> Vll_calculate1/1(V1)
  [V_C] -> Vll_calculate1/2(V2)
  [Short_AB] -> Vll_calculate/3(Fault)
  [Short_BC] -> Vll_calculate1/3(Fault)
  [Short_CA] -> Vll_calculate2/3(Fault)
  [V_BC] -> Mux/2
  [V_CA] -> Mux/3
  [V_AB] -> Mux/1
  Mux/1 -> Vll/1
  V_plus/1 -> Subtract/1, [vdc_plus]
  V_minus/1 -> Subtract/2, [vdc_neg]
  Subtract/1 -> Gain/1
  Gain/1 -> [vdc_half]
  Data Type Conversion/1 -> [Close_Ap]
  Data Type Conversion1/1 -> [Close_Bp]
  Data Type Conversion2/1 -> [Close_Cp]
  Data Type Conversion3/1 -> [Close_An]
  Data Type Conversion4/1 -> [Close_Bn]
  Data Type Conversion5/1 -> [Close_Cn]
  Mux1/1 -> V/1
  [V_A] -> Mux1/1
  [V_C] -> Mux1/3
  [V_B] -> Mux1/2
  ideal_switch_flag/1 -> [ideal_switch_flag]
  [ideal_switch_flag] -> Calculate Phase Voltage/8(Ideal_Switch_Flag)
  [ideal_switch_flag] -> Calculate Phase Voltage1/8(Ideal_Switch_Flag)
  [ideal_switch_flag] -> Calculate Phase Voltage2/8(Ideal_Switch_Flag)
  Calculate Phase Voltage/2(I_DC) -> [I_A_DC]
  Calculate Phase Voltage1/2(I_DC) -> [I_B_DC]
  Calculate Phase Voltage2/2(I_DC) -> [I_C_DC]
  [I_A_DC] -> Add/1
  [I_B_DC] -> Add/2
  [I_C_DC] -> Add/3
  Add/1 -> IDC/1
  Demux/2 -> [An_extern]
  Demux/1 -> [Ap_extern]
  Demux/3 -> [Bp_extern]
  Demux/4 -> [Bn_extern]
  Demux/5 -> [Cp_extern]
  Demux/6 -> [Cn_extern]
  Data Type Conversion12/1 -> Incorporate Fault Signals/16(C-)
  Data Type Conversion13/1 -> Incorporate Fault Signals/10(A-)
  Data Type Conversion15/1 -> Incorporate Fault Signals/13(B-)
  Data Type Conversion14/1 -> Incorporate Fault Signals/7(C+)
  Data Type Conversion16/1 -> Incorporate Fault Signals/4(B+)
  Data Type Conversion17/1 -> Incorporate Fault Signals/1(A+)

== system FOC_BLDC_HIL/Field Oriented Control/Current Controller/Trapezoidal emf estimator/Clark and Park ==
  eabc : Inport
  angle : Inport  Port=2
  Demux : Demux  Outputs=3
  Mux : Mux  Inputs=2
  Mux1 : Mux  Inputs=3
  Mux2 : Mux  Inputs=2
  To calculate Alpha : Fcn  Expr=sqrt(3/2)*u
  To calculate Beta : Fcn  Expr=sqrt(1/2)*(u(1)-u(2))
  To calculate d : Fcn  Expr=u[1]*cos(u[3])-u[2]*sin(u[3])
  To calculate q : Fcn  Expr=u[1]*sin(u[3])+u[2]*cos(u[3])
  edq : Outport  VectorParamsAs1DForOutWhenUnconnected=off
  wires:
  Mux2/1 -> edq/1
  To calculate d/1 -> Mux2/1
  angle/1 -> Mux1/3
  To calculate Beta/1 -> Mux1/2
  To calculate Alpha/1 -> Mux1/1
  To calculate q/1 -> Mux2/2
  Mux1/1 -> To calculate q/1, To calculate d/1
  Mux/1 -> To calculate Beta/1
  Demux/3 -> Mux/2
  Demux/2 -> Mux/1
  Demux/1 -> To calculate Alpha/1
  eabc/1 -> Demux/1

== system FOC_BLDC_HIL/Field Oriented Control/Current Controller/Trapezoidal emf estimator/Emf waveform ==
  Segment : Inport
  angle_el : Inport  Port=2
  -1 : Gain  Gain=-1
  1 : Constant  OutDataTypeStr=single  SampleTime=-1
  2*pi : Constant  Value=2*pi  OutDataTypeStr=single  SampleTime=-1
  2*pi/3 : Constant  Value=2*pi/3  OutDataTypeStr=single  SampleTime=-1
  6/pi : Constant  Value=6/pi  OutDataTypeStr=single  SampleTime=-1
  Add : Sum  Inputs=+-
  Add1 : Sum  Inputs=+-
  Add2 : Sum  Inputs=+-
  Add3 : Sum
  Multiport Switch : MultiPortSwitch  Inputs=4
  Product : Product
  Product1 : Product
  Emf waveform : Outport  VectorParamsAs1DForOutWhenUnconnected=off
  wires:
  Segment/1 -> Multiport Switch/1
  Add2/1 -> Product1/1
  -1/1 -> Multiport Switch/4
  Product/1 -> Add3/2
  6/pi/1 -> Product1/2, Product/1
  Multiport Switch/1 -> Emf waveform/1
  Add3/1 -> Multiport Switch/5
  2*pi/3/1 -> Add2/2
  Add/1 -> Multiport Switch/3
  1/1 -> Add/1, Add3/1, -1/1, Multiport Switch/2
  Product1/1 -> Add/2
  Add1/1 -> Product/2
  2*pi/1 -> Add1/2
  angle_el/1 -> Add2/1, Add1/1

== system FOC_BLDC_HIL/Field Oriented Control/Current Controller/Trapezoidal emf estimator/Segment selector ==
  angle_el : Inport
  1 : Gain
  2 : Gain  Gain=2
  3 : Gain  Gain=3
  4 : Gain  Gain=4
  <2*pi : simulink/Logic and Bit Operations/Compare To Constant  relop=<  const=2*pi  OutDataTypeStr=boolean  ZeroCross=off
  <2*pi/3 : simulink/Logic and Bit Operations/Compare To Constant  relop=<  const=2*pi/3  OutDataTypeStr=boolean  ZeroCross=off
  <5pi/3 : simulink/Logic and Bit Operations/Compare To Constant  relop=<  const=5*pi/3  OutDataTypeStr=boolean  ZeroCross=off
  <pi : simulink/Logic and Bit Operations/Compare To Constant  relop=<  const=pi  OutDataTypeStr=boolean  ZeroCross=off
  >=0 : simulink/Logic and Bit Operations/Compare To Constant  relop=>=  const=0  OutDataTypeStr=boolean  ZeroCross=off
  >=2*pi/3 : simulink/Logic and Bit Operations/Compare To Constant  relop=>=  const=2*pi/3  OutDataTypeStr=boolean  ZeroCross=off
  >=5*pi/3 : simulink/Logic and Bit Operations/Compare To Constant  relop=>=  const=5*pi/3  OutDataTypeStr=boolean  ZeroCross=off
  >=pi : simulink/Logic and Bit Operations/Compare To Constant  relop=>=  const=pi  OutDataTypeStr=boolean  ZeroCross=off
  Add : Sum  Inputs=++++
  Saturation : Saturate  UpperLimit=4  LowerLimit=1
  sector {1..4} (4 alike) : Product
  Segment : Outport  VectorParamsAs1DForOutWhenUnconnected=off
  wires:
  angle_el/1 -> >=5*pi/3/1, <2*pi/1, <5pi/3/1, >=pi/1, <pi/1, >=2*pi/3/1, <2*pi/3/1, >=0/1
  <pi/1 -> sector 2/2
  >=0/1 -> sector 1/1
  sector 3/1 -> 3/1
  sector 2/1 -> 2/1
  sector 4/1 -> 4/1
  <2*pi/1 -> sector 4/2
  >=5*pi/3/1 -> sector 4/1
  >=2*pi/3/1 -> sector 2/1
  sector 1/1 -> 1/1
  <5pi/3/1 -> sector 3/2
  <2*pi/3/1 -> sector 1/2
  >=pi/1 -> sector 3/1
  4/1 -> Add/4
  3/1 -> Add/3
  2/1 -> Add/2
  1/1 -> Add/1
  Add/1 -> Saturation/1
  Saturation/1 -> Segment/1
